simulink model "taller1_simulink_v2"  (R2026a)
settings: Solver=ode45  StopTime=t_final
InitFcn:
  | run('/home/sergio/Escritorio/tdc/taller1_final/init_simulink_v2.m')
values from neighbouring files (symbols this model uses):
  dist_amp = deg2rad(1.0)    [init_simulink.m]    (also in init_simulink_v2.m)
  dist_enabled = 1    [init_simulink_v2.m]
  dist_freq = 2*pi*6    (= 37.6991118431)    [init_simulink.m]    (also in init_simulink_v2.m)
  n_Kphi = size(Kphi_A, 1)    [init_simulink_v2.m]
  n_Ktheta = size(Ktheta_A, 1)    [init_simulink_v2.m]
  n_p = size(Gp_A, 1)    [init_simulink_v2.m]
  n_phi = size(Gphi_A, 1)    [init_simulink_v2.m]
  n_q = size(Gq_A, 1)    [init_simulink_v2.m]
  n_theta = size(Gtheta_A, 1)    [init_simulink_v2.m]
  noise_enabled = 1    [init_simulink_v2.m]
  noise_power_lat = 1e-3    (= 0.001)    [init_simulink.m]    (also in init_simulink_v2.m)
  noise_power_long = 1e-4    (= 0.0001)    [init_simulink.m]    (also in init_simulink_v2.m)
  noise_sample_time = 0.005    [init_simulink.m]    (also in init_simulink_v2.m)
  sas_D_p = kd_phi    (= 0.05)    [init_simulink.m]    (also in init_simulink_v2.m)
  sas_D_q = kd_theta    (= -0.2)    [init_simulink.m]    (also in init_simulink_v2.m)
  t_step = 1.0    (= 1)    [init_simulink.m]    (also in init_simulink_v2.m)
  umax = deg2rad(control_limit_deg)    [init_simulink.m]    (also in init_simulink_v2.m)
undefined symbols (not defined in the file or in its folder): cas_pi_phi_den, cas_pi_phi_num, cas_pi_theta_den, cas_pi_theta_num, Gp_A, Gp_B, Gp_C, Gp_D, Gphi_A, Gphi_B, Gphi_C, Gphi_D, Gq_A, Gq_B, Gq_C, Gq_D, Gtheta_A, Gtheta_B, Gtheta_C, Gtheta_D, Kphi_A, Kphi_B, Kphi_C, Kphi_D, Ktheta_A, Ktheta_B, Ktheta_C, Ktheta_D, Kyaw_A, Kyaw_B, Kyaw_C, Kyaw_D
settings Model: Creator=sergio  LastModifiedBy=sergio

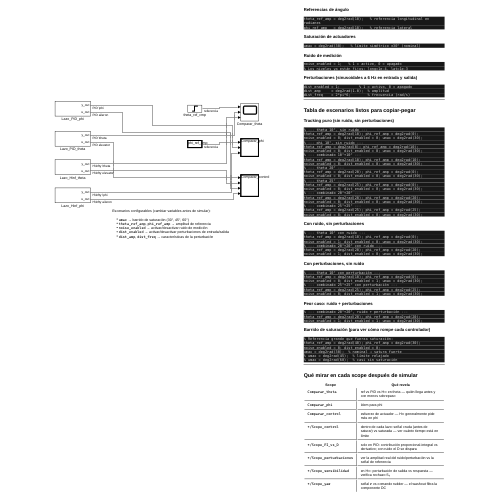
[thumbnail: Simulink's stored preview of the top-level diagram]
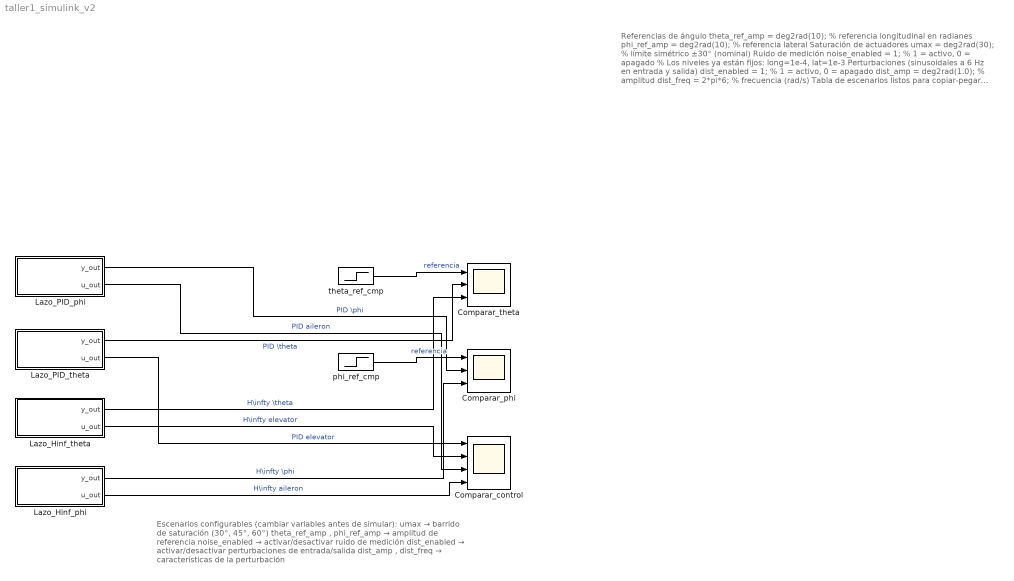
== system taller1_simulink_v2 ==
  note: Referencias de ángulo
      | theta_ref_amp = deg2rad(10); % referencia longitudinal en radianes
      | phi_ref_amp = deg2rad(10); % referencia lateral
      | Saturación de actuadores
      | umax = deg2rad(30); % límite simétrico ±30° (nominal)
      | Ruido de medición
      | noise_enabled = 1; % 1 = activo, 0 = apagado
      | % Los niveles ya están fijos: long=1e-4, lat=1e-3
      | Perturbaciones (sinusoidales a 6 Hz en entrada y salida)
      | dist_enabled = 1; % 1 = activo, 0 = apagado
      | dist_amp = deg2rad(1.0); % amplitud
      | dist_freq = 2*pi*6; % frecuencia (rad/s)
      | Tabla de escenarios listos para copiar-pegar
      | Tracking puro (sin ruido, sin perturbaciones)
      | % --- theta 10°, sin ruido ---
      | theta_ref_amp = deg2rad(10); phi_ref_amp = deg2rad(0);
      | noise_enabled = 0; dist_enabled = 0; umax = deg2rad(30);
      | % --- phi 10°, sin ruido ---
      | theta_ref_amp = deg2rad(0); phi_ref_amp = deg2rad(10);
      | noise_enabled = 0; dist_enabled = 0; umax = deg2rad(30);
      | % --- combinado 10°+10° ---
      | theta_ref_amp = deg2rad(10); phi_ref_amp = deg2rad(10);
      | noise_enabled = 0; dist_enabled = 0; umax = deg2rad(30);
      | % --- theta 20° ---
      | theta_ref_amp = deg2rad(20); phi_ref_amp = deg2rad(0);
      | noise_enabled = 0; dist_enabled = 0; umax = deg2rad(30);
      | % --- theta 25° ---
      | theta_ref_amp = deg2rad(25); phi_ref_amp = deg2rad(0);
      | noise_enabled = 0; dist_enabled = 0; umax = deg2rad(30);
      | % --- combinado 20°+20° ---
      | theta_ref_amp = deg2rad(20); phi_ref_amp = deg2rad(20);
      | noise_enabled = 0; dist_enabled = 0; umax = deg2rad(30);
      | % --- combinado 25°+25° ---
      | theta_ref_amp = deg2rad(25); phi_ref_amp = deg2rad(25);
      | noise_enabled = 0; dist_enabled = 0; umax = deg2rad(30);
      | Con ruido, sin perturbaciones
      | % --- theta 10° con ruido ---
      | theta_ref_amp = deg2rad(10); phi_ref_amp = deg2rad(0);
      | noise_enabled = 1; dist_enabled = 0; umax = deg2rad(30);
      | % --- combinado 20°+20° con ruido ---
      | theta_ref_amp = deg2rad(20); phi_ref_amp = deg2rad(20);
      | noise_enabled = 1; dist_enabled = 0; umax = deg2rad(30);
      | Con perturbaciones, sin ruido
      | % --- theta 10° con perturbación ---
      | theta_ref_amp = deg2rad(10); phi_ref_amp = deg2rad(0);
      | noise_enabled = 0; dist_enabled = 1; umax = deg2rad(30);
      | % --- combinado 25°+25° con perturbación ---
      | theta_ref_amp = deg2rad(25); phi_ref_amp = deg2rad(25);
      | noise_enabled = 0; dist_enabled = 1; umax = deg2rad(30);
      | Peor caso: ruido + perturbaciones
      | % --- combinado 20°+20°, ruido + perturbación ---
      | theta_ref_amp = deg2rad(20); phi_ref_amp = deg2rad(20);
      | noise_enabled = 1; dist_enabled = 1; umax = deg2rad(30);
      | Barrido de saturación (para ver cómo rompe cada controlador)
      | % Referencia grande que fuerza saturación:
      | theta_ref_amp = deg2rad(40); phi_ref_amp = deg2rad(30);
      | noise_enabled = 0; dist_enabled = 0;
      | umax = deg2rad(30); % nominal → satura fuerte
      | % umax = deg2rad(45); % límite relajado
      | % umax = deg2rad(60); % casi sin saturación
      | Qué mirar en cada scope después de simular
      |
      | Scope
      | Qué revela
      |
      | Comparar_theta
      | ref vs PID vs H∞ en theta — quién llega antes y con menos sobrepaso
      |
      | Comparar_phi
      | ídem para phi
      |
      | Comparar_control
      | esfuerzo de actuador — H∞ generalmente pide más en phi
      |
      | */Scope_control
      | dentro de cada lazo: señal cruda (antes de saturar) vs saturada — ver cuánto tiempo está en límite
      |
      | */Scope_PI_vs_D
      | solo en PID: contribución proporcional-integral vs derivativo; con ruido el D se dispara
      |
      | */Scope_perturbaciones
      | ver la amplitud real del ruido/perturbación vs la señal de referencia
      |
      | */Scope_sensibilidad
      | en H∞: perturbación de salida vs respuesta — verifica rechazo S₀
      |
      | */Scope_yaw
      | señal r vs comando rudder — el washout filtra la componente DC
  note: Escenarios configurables (cambiar variables antes de simular):
      | umax → barrido de saturación (30°, 45°, 60°)
      | theta_ref_amp , phi_ref_amp → amplitud de referencia
      | noise_enabled → activar/desactivar ruido de medición
      | dist_enabled → activar/desactivar perturbaciones de entrada/salida
      | dist_amp , dist_freq → características de la perturbación
  Comparar_control : Scope  NumInputPorts=4
      settings: TimeSpan=auto  Title=Comparacion control — PID vs H\infty (elevator y aileron)  ActiveDisplayYMinimum=-1.1700186794974847  ActiveDisplayYMaximum=0.98411739676696031  YLabel=senal [rad]  DataLoggingVariableName=log_cmp_ctrl
  Comparar_phi : Scope  NumInputPorts=3
      settings: TimeSpan=auto  Title=Comparacion \phi — PID vs H\infty  ActiveDisplayYMinimum=-0.55058674297722521  ActiveDisplayYMaximum=4.7705343385250849  YLabel=angulo [rad]  DataLoggingVariableName=log_cmp_phi
  Comparar_theta : Scope  NumInputPorts=3
      settings: TimeSpan=auto  Title=Comparacion \theta — PID vs H\infty  ActiveDisplayYMinimum=-0.029642247335690406  ActiveDisplayYMaximum=0.20027872044110884  YLabel=angulo [rad]  DataLoggingVariableName=log_cmp_theta
  Lazo_Hinf_phi : Subsystem
  Lazo_Hinf_theta : Subsystem
  Lazo_PID_phi : Subsystem
  Lazo_PID_theta : Subsystem
  phi_ref_cmp : Step  Time=t_step  FinalValue=phi_ref_amp  SampleTime=0
  theta_ref_cmp : Step  Time=t_step  FinalValue=theta_ref_amp  SampleTime=0
  wires:
  theta_ref_cmp/1 -> Comparar_theta/1  "referencia"
  Lazo_PID_theta/1(y_out) -> Comparar_theta/2  "PID \\theta"
  Lazo_Hinf_theta/1(y_out) -> Comparar_theta/3  "H\\infty \\theta"
  phi_ref_cmp/1 -> Comparar_phi/1  "referencia"
  Lazo_PID_phi/1(y_out) -> Comparar_phi/2  "PID \\phi"
  Lazo_Hinf_phi/1(y_out) -> Comparar_phi/3  "H\\infty \\phi"
  Lazo_PID_theta/2(u_out) -> Comparar_control/1  "PID elevator"
  Lazo_Hinf_theta/2(u_out) -> Comparar_control/2  "H\\infty elevator"
  Lazo_PID_phi/2(u_out) -> Comparar_control/3  "PID aileron"
  Lazo_Hinf_phi/2(u_out) -> Comparar_control/4  "H\\infty aileron"

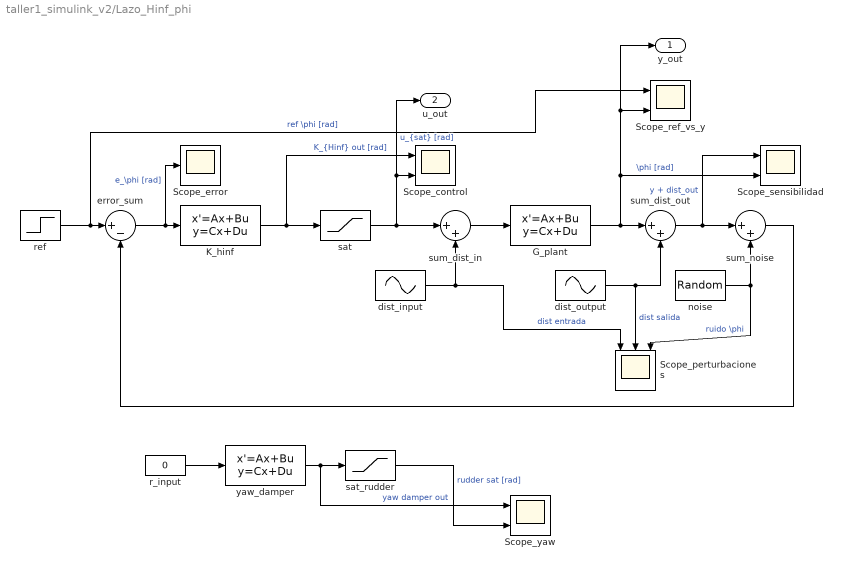
== system taller1_simulink_v2/Lazo_Hinf_phi ==
  G_plant : StateSpace  A=Gphi_A  B=Gphi_B  C=Gphi_C  D=Gphi_D  InitialCondition=zeros(n_phi,1)
  K_hinf : StateSpace  A=Kphi_A  B=Kphi_B  C=Kphi_C  D=Kphi_D  InitialCondition=zeros(n_Kphi,1)
  Scope_control : Scope  NumInputPorts=2
      settings: TimeSpan=auto  Title=H\infty \phi — Senal de control (cruda vs saturada)  YLabel=aileron [rad]  DataLoggingVariableName=log_hinf_phi_u
  Scope_error : Scope
      settings: TimeSpan=auto  Title=H\infty \phi — Error de seguimiento  YLabel=error [rad]  DataLoggingVariableName=log_hinf_phi_e
  Scope_perturbaciones : Scope  NumInputPorts=3
      settings: TimeSpan=auto  Title=H\infty \phi — Perturbaciones y ruido  YLabel=magnitud
  Scope_ref_vs_y : Scope  NumInputPorts=2
      settings: TimeSpan=auto  Title=H\infty \phi — Seguimiento de referencia  YLabel=angulo [rad]  DataLoggingVariableName=log_hinf_phi_y
  Scope_sensibilidad : Scope  NumInputPorts=2
      settings: TimeSpan=auto  Title=H\infty \phi — Rechazo de perturbacion de salida (S_0)  YLabel=angulo [rad]
  Scope_yaw : Scope  NumInputPorts=2
      settings: TimeSpan=auto  Title=H\infty \phi — Yaw damper (salida y saturacion)  YLabel=rudder [rad]
  dist_input : Sin  Amplitude=dist_amp*dist_enabled  Frequency=dist_freq  SampleTime=0
  dist_output : Sin  Amplitude=dist_amp*dist_enabled*0.5  Frequency=dist_freq*1.5  SampleTime=0
  error_sum : Sum  Inputs=|+-
  noise : RandomNumber  Variance=noise_power_lat*noise_enabled  Seed=13  SampleTime=noise_sample_time
  r_input : Constant  Value=0
  ref : Step  Time=t_step  FinalValue=phi_ref_amp  SampleTime=0
  sat : Saturate  UpperLimit=umax  LowerLimit=-umax
  sat_rudder : Saturate  UpperLimit=umax  LowerLimit=-umax
  sum_dist_in : Sum  Inputs=|++
  sum_dist_out : Sum  Inputs=|++
  sum_noise : Sum  Inputs=|++
  yaw_damper : StateSpace  A=Kyaw_A  B=Kyaw_B  C=Kyaw_C  D=Kyaw_D  InitialCondition=0
  y_out : Outport
  u_out : Outport  Port=2
  wires:
  ref/1 -> Scope_ref_vs_y/1, error_sum/1  "ref \\phi [rad]"
  error_sum/1 -> Scope_error/1, K_hinf/1  "e_\\phi [rad]"
  K_hinf/1 -> sat/1, Scope_control/1  "K_{Hinf} out [rad]"
  sat/1 -> u_out/1, Scope_control/2, sum_dist_in/1  "u_{sat} [rad]"
  dist_input/1 -> sum_dist_in/2, Scope_perturbaciones/1  "dist entrada"
  sum_dist_in/1 -> G_plant/1
  G_plant/1 -> y_out/1, Scope_ref_vs_y/2, Scope_sensibilidad/2, sum_dist_out/1  "\\phi [rad]"
  dist_output/1 -> sum_dist_out/2, Scope_perturbaciones/2  "dist salida"
  sum_dist_out/1 -> sum_noise/1, Scope_sensibilidad/1  "y + dist_out"
  noise/1 -> sum_noise/2, Scope_perturbaciones/3  "ruido \\phi"
  sum_noise/1 -> error_sum/2
  r_input/1 -> yaw_damper/1
  yaw_damper/1 -> sat_rudder/1, Scope_yaw/1  "yaw damper out"
  sat_rudder/1 -> Scope_yaw/2  "rudder sat [rad]"

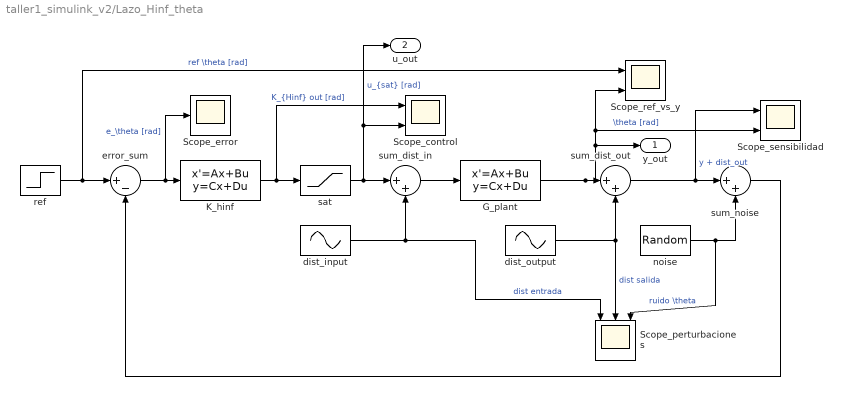
== system taller1_simulink_v2/Lazo_Hinf_theta ==
  G_plant : StateSpace  A=Gtheta_A  B=Gtheta_B  C=Gtheta_C  D=Gtheta_D  InitialCondition=zeros(n_theta,1)
  K_hinf : StateSpace  A=Ktheta_A  B=Ktheta_B  C=Ktheta_C  D=Ktheta_D  InitialCondition=zeros(n_Ktheta,1)
  Scope_control : Scope  NumInputPorts=2
      settings: TimeSpan=auto  Title=H\infty \theta — Senal de control (cruda vs saturada)  YLabel=elevator [rad]  DataLoggingVariableName=log_hinf_theta_u
  Scope_error : Scope
      settings: TimeSpan=auto  Title=H\infty \theta — Error de seguimiento  YLabel=error [rad]  DataLoggingVariableName=log_hinf_theta_e
  Scope_perturbaciones : Scope  NumInputPorts=3
      settings: TimeSpan=auto  Title=H\infty \theta — Perturbaciones y ruido  YLabel=magnitud
  Scope_ref_vs_y : Scope  NumInputPorts=2
      settings: TimeSpan=auto  Title=H\infty \theta — Seguimiento de referencia  YLabel=angulo [rad]  DataLoggingVariableName=log_hinf_theta_y
  Scope_sensibilidad : Scope  NumInputPorts=2
      settings: TimeSpan=auto  Title=H\infty \theta — Rechazo de perturbacion de salida (S_0)  YLabel=angulo [rad]
  dist_input : Sin  Amplitude=dist_amp*dist_enabled  Frequency=dist_freq  SampleTime=0
  dist_output : Sin  Amplitude=dist_amp*dist_enabled*0.5  Frequency=dist_freq*1.5  SampleTime=0
  error_sum : Sum  Inputs=|+-
  noise : RandomNumber  Variance=noise_power_long*noise_enabled  Seed=13  SampleTime=noise_sample_time
  ref : Step  Time=t_step  FinalValue=theta_ref_amp  SampleTime=0
  sat : Saturate  UpperLimit=umax  LowerLimit=-umax
  sum_dist_in : Sum  Inputs=|++
  sum_dist_out : Sum  Inputs=|++
  sum_noise : Sum  Inputs=|++
  y_out : Outport
  u_out : Outport  Port=2
  wires:
  ref/1 -> error_sum/1, Scope_ref_vs_y/1  "ref \\theta [rad]"
  error_sum/1 -> Scope_error/1, K_hinf/1  "e_\\theta [rad]"
  K_hinf/1 -> Scope_control/1, sat/1  "K_{Hinf} out [rad]"
  sat/1 -> u_out/1, Scope_control/2, sum_dist_in/1  "u_{sat} [rad]"
  dist_input/1 -> Scope_perturbaciones/1, sum_dist_in/2  "dist entrada"
  sum_dist_in/1 -> G_plant/1
  G_plant/1 -> Scope_ref_vs_y/2, Scope_sensibilidad/2, y_out/1, sum_dist_out/1  "\\theta [rad]"
  dist_output/1 -> sum_dist_out/2, Scope_perturbaciones/2  "dist salida"
  sum_dist_out/1 -> Scope_sensibilidad/1, sum_noise/1  "y + dist_out"
  noise/1 -> sum_noise/2, Scope_perturbaciones/3  "ruido \\theta"
  sum_noise/1 -> error_sum/2

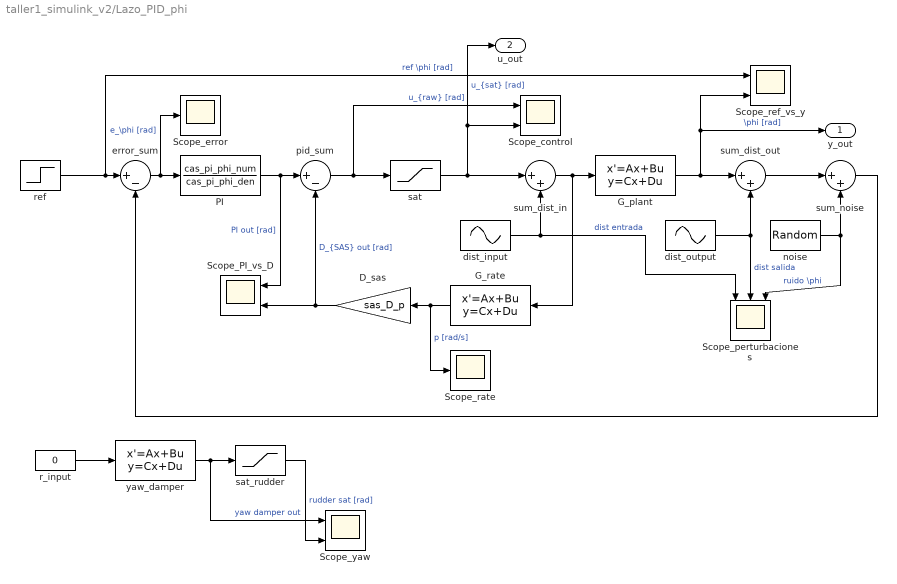
== system taller1_simulink_v2/Lazo_PID_phi ==
  D_sas : Gain  Gain=sas_D_p
  G_plant : StateSpace  A=Gphi_A  B=Gphi_B  C=Gphi_C  D=Gphi_D  InitialCondition=zeros(n_phi,1)
  G_rate : StateSpace  A=Gp_A  B=Gp_B  C=Gp_C  D=Gp_D  InitialCondition=zeros(n_p,1)
  PI : TransferFcn  Numerator=cas_pi_phi_num  Denominator=cas_pi_phi_den
  Scope_PI_vs_D : Scope  NumInputPorts=2
      settings: TimeSpan=auto  Title=PID \phi — Contribucion PI vs D_{SAS}  YLabel=magnitud [rad]
  Scope_control : Scope  NumInputPorts=2
      settings: TimeSpan=auto  Title=PID \phi — Senal de control (cruda vs saturada)  YLabel=aileron [rad]  DataLoggingVariableName=log_pid_phi_u
  Scope_error : Scope
      settings: TimeSpan=auto  Title=PID \phi — Error de seguimiento  ActiveDisplayYMinimum=-1.3301704294745242  ActiveDisplayYMaximum=4.02561658247627  YLabel=error [rad]  DataLoggingVariableName=log_pid_phi_e
  Scope_perturbaciones : Scope  NumInputPorts=3
      settings: TimeSpan=auto  Title=PID \phi — Perturbaciones y ruido  YLabel=magnitud
  Scope_rate : Scope
      settings: TimeSpan=auto  Title=PID \phi — Tasa de alabeo p  YLabel=p [rad/s]
  Scope_ref_vs_y : Scope  NumInputPorts=2
      settings: TimeSpan=auto  Title=PID \phi — Seguimiento de referencia  ActiveDisplayYMinimum=-0.53837497126202039  ActiveDisplayYMaximum=4.7691774750011735  YLabel=angulo [rad]  DataLoggingVariableName=log_pid_phi_y
  Scope_yaw : Scope  NumInputPorts=2
      settings: TimeSpan=auto  Title=PID \phi — Yaw damper (salida y saturacion)  YLabel=rudder [rad]
  dist_input : Sin  Amplitude=dist_amp*dist_enabled  Frequency=dist_freq  SampleTime=0
  dist_output : Sin  Amplitude=dist_amp*dist_enabled*0.5  Frequency=dist_freq*1.5  SampleTime=0
  error_sum : Sum  Inputs=|+-
  noise : RandomNumber  Variance=noise_power_lat*noise_enabled  Seed=11  SampleTime=noise_sample_time
  pid_sum : Sum  Inputs=|+-
  r_input : Constant  Value=0
  ref : Step  Time=t_step  FinalValue=phi_ref_amp  SampleTime=0
  sat : Saturate  UpperLimit=umax  LowerLimit=-umax
  sat_rudder : Saturate  UpperLimit=umax  LowerLimit=-umax
  sum_dist_in : Sum  Inputs=|++
  sum_dist_out : Sum  Inputs=|++
  sum_noise : Sum  Inputs=|++
  yaw_damper : StateSpace  A=Kyaw_A  B=Kyaw_B  C=Kyaw_C  D=Kyaw_D  InitialCondition=0
  y_out : Outport
  u_out : Outport  Port=2
  wires:
  ref/1 -> Scope_ref_vs_y/1, error_sum/1  "ref \\phi [rad]"
  error_sum/1 -> PI/1, Scope_error/1  "e_\\phi [rad]"
  PI/1 -> pid_sum/1, Scope_PI_vs_D/1  "PI out [rad]"
  D_sas/1 -> pid_sum/2, Scope_PI_vs_D/2  "D_{SAS} out [rad]"
  pid_sum/1 -> sat/1, Scope_control/1  "u_{raw} [rad]"
  sat/1 -> sum_dist_in/1, u_out/1, Scope_control/2  "u_{sat} [rad]"
  dist_input/1 -> sum_dist_in/2, Scope_perturbaciones/1  "dist entrada"
  sum_dist_in/1 -> G_plant/1, G_rate/1
  G_rate/1 -> Scope_rate/1, D_sas/1  "p [rad/s]"
  G_plant/1 -> y_out/1, Scope_ref_vs_y/2, sum_dist_out/1  "\\phi [rad]"
  dist_output/1 -> sum_dist_out/2, Scope_perturbaciones/2  "dist salida"
  sum_dist_out/1 -> sum_noise/1
  noise/1 -> sum_noise/2, Scope_perturbaciones/3  "ruido \\phi"
  sum_noise/1 -> error_sum/2
  r_input/1 -> yaw_damper/1
  yaw_damper/1 -> Scope_yaw/1, sat_rudder/1  "yaw damper out"
  sat_rudder/1 -> Scope_yaw/2  "rudder sat [rad]"

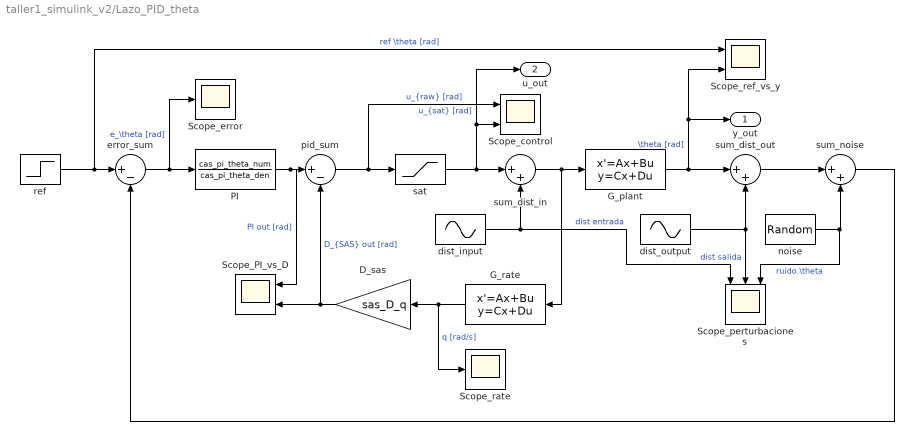
== system taller1_simulink_v2/Lazo_PID_theta ==
  D_sas : Gain  Gain=sas_D_q
  G_plant : StateSpace  A=Gtheta_A  B=Gtheta_B  C=Gtheta_C  D=Gtheta_D  InitialCondition=zeros(n_theta,1)
  G_rate : StateSpace  A=Gq_A  B=Gq_B  C=Gq_C  D=Gq_D  InitialCondition=zeros(n_q,1)
  PI : TransferFcn  Numerator=cas_pi_theta_num  Denominator=cas_pi_theta_den
  Scope_PI_vs_D : Scope  NumInputPorts=2
      settings: TimeSpan=auto  Title=PID \theta — Contribucion PI vs D_{SAS}  YLabel=magnitud [rad]
  Scope_control : Scope  NumInputPorts=2
      settings: TimeSpan=auto  Title=PID \theta — Senal de control (cruda vs saturada)  YLabel=elevator [rad]  DataLoggingVariableName=log_pid_theta_u
  Scope_error : Scope
      settings: TimeSpan=auto  Title=PID \theta — Error de seguimiento  YLabel=error [rad]  DataLoggingVariableName=log_pid_theta_e
  Scope_perturbaciones : Scope  NumInputPorts=3
      settings: TimeSpan=auto  Title=PID \theta — Perturbaciones y ruido  YLabel=magnitud
  Scope_rate : Scope
      settings: TimeSpan=auto  Title=PID \theta — Tasa de cabeceo q  YLabel=q [rad/s]
  Scope_ref_vs_y : Scope  NumInputPorts=2
      settings: TimeSpan=auto  Title=PID \theta — Seguimiento de referencia  YLabel=angulo [rad]  DataLoggingVariableName=log_pid_theta_y
  dist_input : Sin  Amplitude=dist_amp*dist_enabled  Frequency=dist_freq  SampleTime=0
  dist_output : Sin  Amplitude=dist_amp*dist_enabled*0.5  Frequency=dist_freq*1.5  SampleTime=0
  error_sum : Sum  Inputs=|+-
  noise : RandomNumber  Variance=noise_power_long*noise_enabled  Seed=11  SampleTime=noise_sample_time
  pid_sum : Sum  Inputs=|+-
  ref : Step  Time=t_step  FinalValue=theta_ref_amp  SampleTime=0
  sat : Saturate  UpperLimit=umax  LowerLimit=-umax
  sum_dist_in : Sum  Inputs=|++
  sum_dist_out : Sum  Inputs=|++
  sum_noise : Sum  Inputs=|++
  y_out : Outport
  u_out : Outport  Port=2
  wires:
  ref/1 -> error_sum/1, Scope_ref_vs_y/1  "ref \\theta [rad]"
  error_sum/1 -> PI/1, Scope_error/1  "e_\\theta [rad]"
  PI/1 -> Scope_PI_vs_D/1, pid_sum/1  "PI out [rad]"
  D_sas/1 -> pid_sum/2, Scope_PI_vs_D/2  "D_{SAS} out [rad]"
  pid_sum/1 -> sat/1, Scope_control/1  "u_{raw} [rad]"
  sat/1 -> sum_dist_in/1, Scope_control/2, u_out/1  "u_{sat} [rad]"
  dist_input/1 -> Scope_perturbaciones/1, sum_dist_in/2  "dist entrada"
  sum_dist_in/1 -> G_plant/1, G_rate/1
  G_rate/1 -> Scope_rate/1, D_sas/1  "q [rad/s]"
  G_plant/1 -> sum_dist_out/1, y_out/1, Scope_ref_vs_y/2  "\\theta [rad]"
  dist_output/1 -> sum_dist_out/2, Scope_perturbaciones/2  "dist salida"
  sum_dist_out/1 -> sum_noise/1
  noise/1 -> sum_noise/2, Scope_perturbaciones/3  "ruido \\theta"
  sum_noise/1 -> error_sum/2
